simulink library "synths"  (R2012b)
settings: Solver=ode45  StartTime=0.0  StopTime=10.0  RelTol=1e-3
libraries: xbsIndex_r4 x9, xps_library x1
settings Model: Creator=anyoung  LastModifiedBy=ayoung

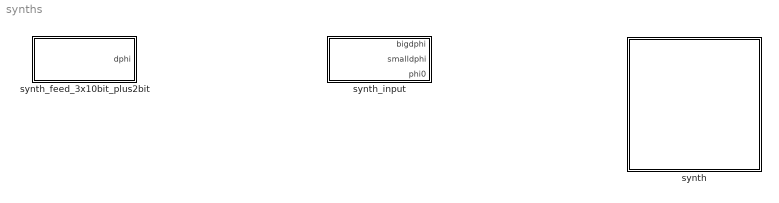
== system synths ==
  synth : Subsystem  mask(synth){n_parout=0, sum_latency=1, n_ph_bits=8, n_amp_bits=8, out_type=Sine and Cosine}
      mask prompts: n_parout "Number of parallel outputs"; sum_latency "Latency (sum)"; n_ph_bits "Bitwidth phase"; n_amp_bits "Bitwidth amplitude"; out_type "Requested outputs"
      mask help:
      | Implements a DDS with demuxed output and reconfigurable phase and frequency.
      |
      | Number of parallel outputs should be at least 2.
      |
      | Adder latencies can be specified, and the overall latency of the DDS is displayed.
      mask init:
      | synth_init(gcb,...
      | 'n_parout',n_parout,...
      | 'sum_latency',sum_latency,...
      | 'n_ph_bits',n_ph_bits,...
      | 'n_amp_bits',n_amp_bits,...
      | 'out_type',out_type ...
      | );
      mask Help: Nothing here yet.
      mask TypeOptions out_type: Sine and Cosine | Sine | Cosine
  synth_feed_3x10bit_plus2bit : Subsystem  mask(synth_feed_3x10bit_plus2bit){dphi=0, demux_dphi=0, phi0=0}
      mask prompts: dphi "Phase increment per sample"; demux_dphi "Phase increment per demux set"; phi0 "Phase offset"
      mask help:
      | Provides simulated input to synth_input register.
      |
      | Three 10bit fields:
      |     dphi: Phase increment between consecutive samples
      |     demux_dphi: Phase increment between consecutive sets of demuxed input
      |     phi0: Phase offset
      |
      | The most-significant 2bit is set to zero.
      mask init:
      | set_param([gcb '/bigdphi'],'const',get_param(gcb,'demux_dphi'));
      | set_param([gcb '/smalldphi'],'const',get_param(gcb,'dphi'));
      | set_param([gcb '/phi0'],'const',get_param(gcb,'phi0'));
  synth_input : Subsystem  mask(synth_input){io_delay=0, sim_in=off, dphi=0, demux_dphi=0, phi0=0}
      mask prompts: io_delay "I/O delay"; sim_in "Sim input?"; dphi "Phase increment per sample"; demux_dphi "Phase increment per demux set"; phi0 "Phase offset"
      mask help:
      | Defines input for synth using a single 32bit software register.
      |
      | I/O delay and optional simulated input for the register are configurable.
      |
      | If simulated input is set, a feed is internally generated using the given parameters for phase increment and offset.
      mask init:
      | synth_input_init(gcb,...
      |     'io_delay',io_delay,...
      |     'sim_in',sim_in,...
      |     'dphi',dphi,...
      |     'demux_dphi',demux_dphi,...
      |     'phi0',phi0);
      mask Callback sim_in:
      | if strcmpi(get_param(gcb,'sim_in'),'on')
      |     set_param(gcb,'MaskEnables',{'on';'on';'on';'on';'on'});
      | else
      |     set_param(gcb,'MaskEnables',{'on';'on';'off';'off';'off'});
      | end

== system synths/synth ==

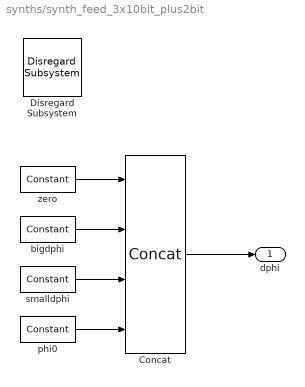
== system synths/synth_feed_3x10bit_plus2bit ==
  Concat : xbsIndex_r4/Concat  num_inputs=4  dbl_ovrd=off  block_type=concat
  Disregard Subsystem : xbsIndex_r4/Disregard Subsystem  Tag=discardX  block_type=disregard
  bigdphi : xbsIndex_r4/Constant  const=0  gui_display_data_type=Fixed-point  arith_type=Unsigned  n_bits=10  bin_pt=0  preci_type=Single  exp_width=8  frac_width=24  explicit_period=on  period=1  equ=P=C  opselect=C  inp2=PCIN>>17  opr=+  inp1=P  carry=CIN  dbl_ovrd=off  block_type=constant
  phi0 : xbsIndex_r4/Constant  const=0  gui_display_data_type=Fixed-point  arith_type=Unsigned  n_bits=10  bin_pt=0  preci_type=Single  exp_width=8  frac_width=24  explicit_period=on  period=1  equ=P=C  opselect=C  inp2=PCIN>>17  opr=+  inp1=P  carry=CIN  dbl_ovrd=off  block_type=constant
  smalldphi : xbsIndex_r4/Constant  const=0  gui_display_data_type=Fixed-point  arith_type=Unsigned  n_bits=10  bin_pt=0  preci_type=Single  exp_width=8  frac_width=24  explicit_period=on  period=1  equ=P=C  opselect=C  inp2=PCIN>>17  opr=+  inp1=P  carry=CIN  dbl_ovrd=off  block_type=constant
  zero : xbsIndex_r4/Constant  const=0  gui_display_data_type=Fixed-point  arith_type=Unsigned  n_bits=2  bin_pt=0  preci_type=Single  exp_width=8  frac_width=24  explicit_period=on  period=1  equ=P=C  opselect=C  inp2=PCIN>>17  opr=+  inp1=P  carry=CIN  dbl_ovrd=off  block_type=constant
  dphi : Outport
  wires:
  Concat/1 -> dphi/1
  zero/1 -> Concat/1
  smalldphi/1 -> Concat/3
  bigdphi/1 -> Concat/2
  phi0/1 -> Concat/4

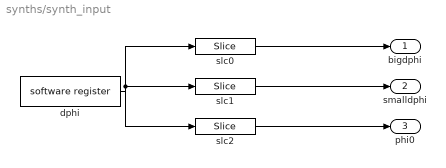
== system synths/synth_input ==
  dphi : xps_library/software register  Tag=xps:sw_reg  mode=one value  io_dir=From Processor  io_delay=0  sample_period=1  names=reg  bitwidths=32  arith_types=0  bin_pts=0  sim_port=off  show_format=off
      settings: AttributesFormatString=1input
  slc0 : xbsIndex_r4/Slice  nbits=10  boolean_output=off  mode=Lower Bit Location + Width  bit1=0  base1=MSB of Input  bit0=20  base0=LSB of Input  dbl_ovrd=off  block_type=slice
  slc1 : xbsIndex_r4/Slice  nbits=10  boolean_output=off  mode=Lower Bit Location + Width  bit1=0  base1=MSB of Input  bit0=10  base0=LSB of Input  dbl_ovrd=off  block_type=slice
  slc2 : xbsIndex_r4/Slice  nbits=10  boolean_output=off  mode=Lower Bit Location + Width  bit1=0  base1=MSB of Input  bit0=0  base0=LSB of Input  dbl_ovrd=off  block_type=slice
  bigdphi : Outport
  smalldphi : Outport  Port=2
  phi0 : Outport  Port=3
  wires:
  dphi/1 -> slc0/1, slc1/1, slc2/1
  slc0/1 -> bigdphi/1
  slc1/1 -> smalldphi/1
  slc2/1 -> phi0/1
